simulink model "Basic_FNPLL"  (R2023a)
settings: Solver=VariableStepAuto  StartTime=0.0  StopTime=1.501e-03  MaxStep=1/(20e9)  RelTol=1e-3
model workspace (MAT data in the model file):
  PhaseNoise_9 = [-44.9660791591 -81.4644293672 -95.4502889633 -100.309141763 -117.548729939]
  PnFrequencyOffset_9 = [10000 100000 1000000 10000000 100000000]
  uniqueString_9 = '81_4724'
libraries: msbPllFoundation x5, msbPllMeasurements x1
settings Model: Creator=osadamasaru  LastModifiedBy=osadamasaru
settings OptimizationCC: ReuseModelBlockBuffer=off

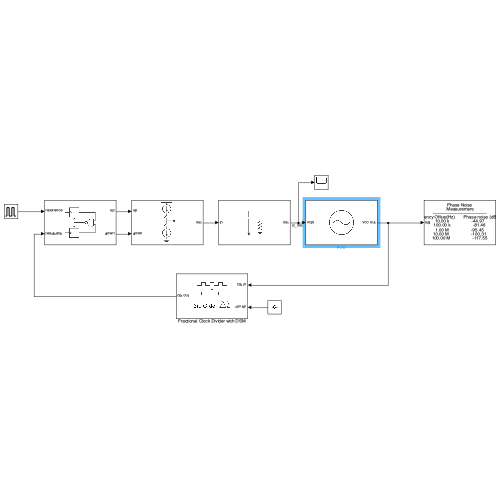
[thumbnail: Simulink's stored preview of the top-level diagram]
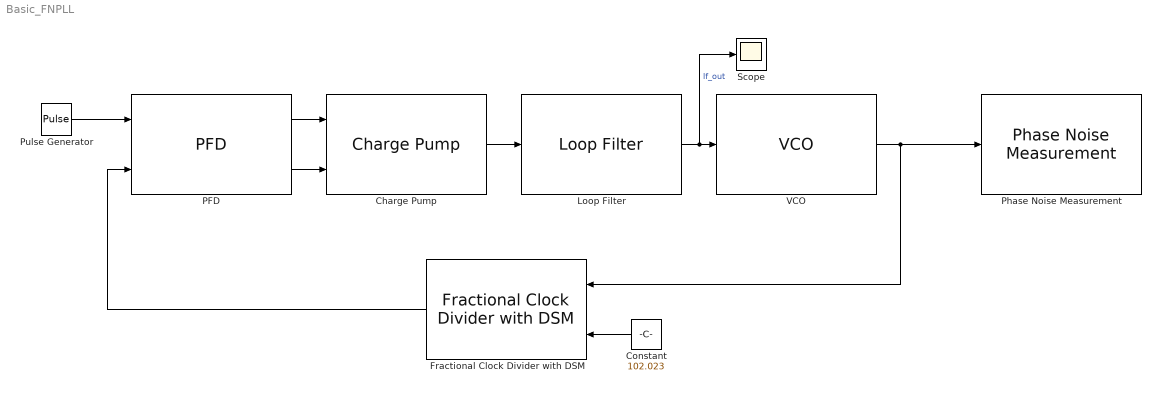
== system Basic_FNPLL ==
  Charge Pump : msbPllFoundation/Charge Pump  OutputCurrent=20e-6  InputThreshold=0.5  ExtraBuffer=off  NBuffer=10  EnableCurrentImpairments=off  CurrentImbalance=1e-7  LeakageCurrent=1e-8  EnableTimingImpairments=off  DefaultOrAdvanced=Default  MaxFreqInterest=10e9  RiseFallUp=5e-9  PropDelayUp=6e-9  RiseFallDown=2e-9  PropDelayDown=4e-9
  Constant : Constant  Value=102.023
  Fractional Clock Divider with DSM : msbPllFoundation/Fractional Clock Divider with DSM  dsm=3rd order  ExtraBuffer=off  NBuffer=1
  Loop Filter : msbPllFoundation/Loop Filter  FilterType=2nd order passive  C1=50.7e-15  C2=456e-15  C3=1.0452e-15  C4=1e-12  R2=1.05e6  R3=51.0435e6  R4=12e3  ExtraBuffer=off  NBuffer=1000  EnableImpairments=off  Temperature=30
  PFD : msbPllFoundation/PFD  DeadbandCompensation=30e-12  ExtraBuffer=off  NBuffer=10  EnableImpairments=off  DefaultOrAdvanced=Default  MaxFreqInterest=10e9  RiseFallTime=30e-12  PropDelay=50e-12
  Phase Noise Measurement : msbPllMeasurements/Phase Noise Measurement  SampleRate=21.6e9  ResBandwidth=10e3  SpectralAverages=10  HoldOffTime=1e-6  PhaseNoiseFreqOffset=[10e3 100e3 1e6 10e6 100e6]  SpecifyTarget=off  TargetPhaseNoise=[-300 -300 -300 -300 -300]  ExtraBuffer=off  NBuffer=10
  Pulse Generator : DiscretePulseGenerator  PulseType=Time based  Period=1/(20e6)  PulseWidth=50
  Scope : Scope
  VCO : msbPllFoundation/VCO  SpecifyUsing=Voltage sensitivity  Kvco=30e6  Fo=2e9  ControlVoltage=[-5 0 5]  OutputFrequency=[2e9 2.5e9 3e9]  Amplitude=1  ExtraBuffer=off  NBuffer=10  AddPhaseNoise=on  Foffset=[30e3 100e3 1e6 3e6 10e6]  PhaseNoise=[-56 -106 -132 -143 -152]  MaxKvco=30000000
  wires:
  Loop Filter/1 -> Scope/1, VCO/1  "lf_out"
  Charge Pump/1 -> Loop Filter/1
  PFD/1 -> Charge Pump/1
  PFD/2 -> Charge Pump/2
  VCO/1 -> Phase Noise Measurement/1, Fractional Clock Divider with DSM/1
  Fractional Clock Divider with DSM/1 -> PFD/2
  Constant/1 -> Fractional Clock Divider with DSM/2
  Pulse Generator/1 -> PFD/1
